simulink model "Torque_Control_Test"  (R2026a)
settings: Solver=VariableStepAuto  StopTime=2
undefined symbols (not defined in the file): Iq_max, K_t2iq

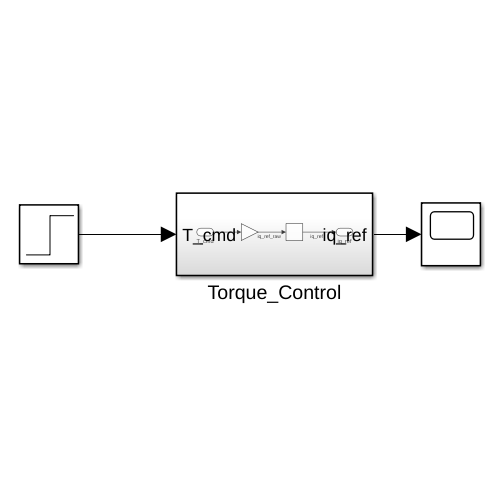
[thumbnail: Simulink's stored preview of the top-level diagram]
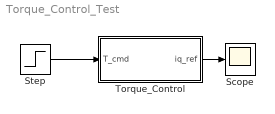
== system Torque_Control_Test ==
  Scope : Scope
      settings: ActiveDisplayYMinimum=1.8518518518518521  ActiveDisplayYMaximum=20.370370370370367
  Step : Step  Time=0.1  InitialValue=1  FinalValue=5  SampleTime=0
  Torque_Control : Subsystem
  wires:
  Step/1 -> Torque_Control/1(T_cmd)
  Torque_Control/1(iq_ref) -> Scope/1

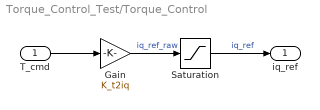
== system Torque_Control_Test/Torque_Control ==
  T_cmd : Inport
  Gain : Gain  Gain=K_t2iq
  Saturation : Saturate  UpperLimit=Iq_max  LowerLimit=-Iq_max
  iq_ref : Outport
  wires:
  T_cmd/1 -> Gain/1
  Gain/1 -> Saturation/1  "iq_ref_raw"
  Saturation/1 -> iq_ref/1  "iq_ref"
